simulink model "DSimulator_robotPRR_KB_NPC"  (Simulink 9.0)
settings: Solver=ode1  StartTime=0.0  StopTime=40.0  FixedStep=0.01  RelTol=1e-3  EnableMultiTasking=on
undefined symbols (not defined in the file or in its folder): Dinamic_robotPRR_KB, SimpleRobotPlot
settings Model: SuppressorTable=22 serialization::archive 11 0 6 0 0 0 11 0  Creator=E. Dean  LastModifiedBy=nirnai  SimulationMode=accelerator
settings DataIOCC: LimitDataPoints=on  SignalLoggingSaveFormat=ModelDataLogs
settings OptimizationCC: ExpressionDepthLimit=2147483647
settings DebuggingCC: SolverPrmCheckMsg=warning  FcnCallInpInsideContextMsg=warning  StateNameClashWarn=warning
settings GRTTargetCC: GeneratePreprocessorConditionals=Disable all  CombineOutputUpdateFcns=off  GRTInterface=on

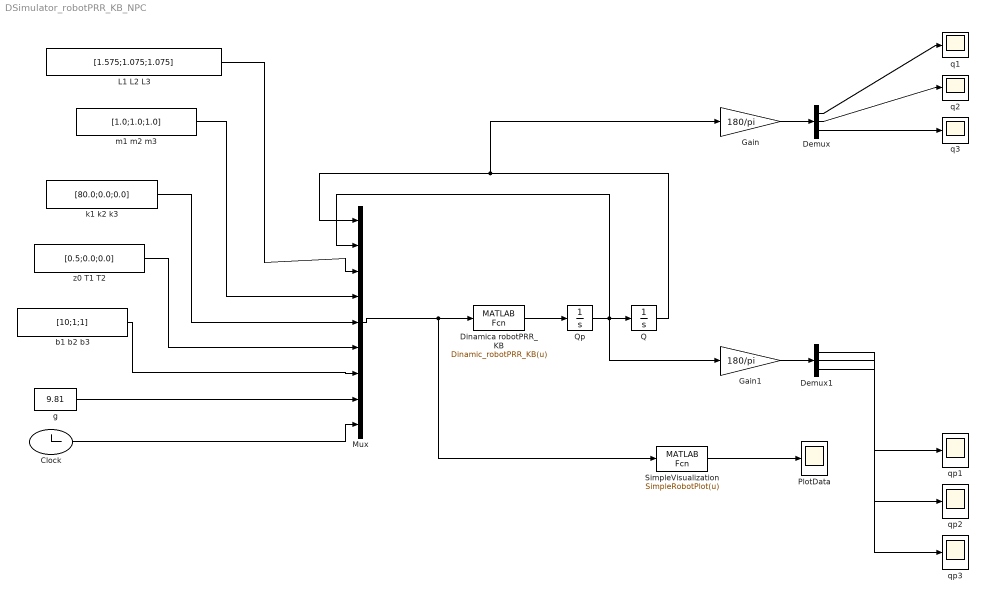
== system DSimulator_robotPRR_KB_NPC ==
  " L1 L2 L3 " : Constant  Value=[1.575;1.075;1.075]
  Clock : Clock
  Demux : Demux  Outputs=3
  Demux1 : Demux  Outputs=3
  Dinamica robotPRR_KB : MATLABFcn  MATLABFcn=Dinamic_robotPRR_KB(u)  OutputDimensions=3
  Gain : Gain  Gain=180/pi
  Gain1 : Gain  Gain=180/pi
  Mux : Mux  Inputs=9
  PlotData : Scope
  Q : Integrator  InitialCondition=[0;pi/2;0]  UpperSaturationLimit=[0.5;inf;inf]  LowerSaturationLimit=[-0.5;-inf;-inf]
  Qp : Integrator  InitialCondition=[0;0;0]
  SimpleVisualization : MATLABFcn  MATLABFcn=SimpleRobotPlot(u)  OutputDimensions=3
  "b1 b2 b3 " : Constant  Value=[10;1;1]
  g : Constant  Value=9.81
  k1 k2 k3 : Constant  Value=[80.0;0.0;0.0]
  "m1 m2 m3 " : Constant  Value=[1.0;1.0;1.0]
  q1 : Scope
  q2 : Scope
  q3 : Scope
  qp1 : Scope
  qp2 : Scope
  qp3 : Scope
  z0 T1 T2 : Constant  Value=[0.5;0.0;0.0]
  wires:
  Qp/1 -> Mux/2, Q/1, Gain1/1
  Dinamica robotPRR_KB/1 -> Qp/1
  Q/1 -> Gain/1, Mux/1
  Gain/1 -> Demux/1
  Demux/1 -> q1/1
  Demux/2 -> q2/1
  Demux/3 -> q3/1
  Gain1/1 -> Demux1/1
  Demux1/1 -> qp1/1
  Demux1/2 -> qp2/1
  Demux1/3 -> qp3/1
  " L1 L2 L3 "/1 -> Mux/3
  "m1 m2 m3 "/1 -> Mux/4
  g/1 -> Mux/8
  Clock/1 -> Mux/9
  "b1 b2 b3 "/1 -> Mux/7
  SimpleVisualization/1 -> PlotData/1
  k1 k2 k3/1 -> Mux/5
  Mux/1 -> SimpleVisualization/1, Dinamica robotPRR_KB/1
  z0 T1 T2/1 -> Mux/6
